simulink model "WaterProp"  (Simulink 7.9)
settings: Solver=FixedStepDiscrete  StartTime=0.0  StopTime=stop  FixedStep=1  MaxStep=1  RelTol=1e-3
settings Model: Creator=awohlfei  LastModifiedBy=awohlfei
settings DataIOCC: SaveTime=off

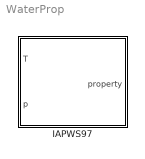
== system WaterProp ==
  IAPWS97 : Subsystem  mask{PROPERTY=DENSITY}
      mask StyleString: popup(DENSITY|HEAT_CAPACITY|THERMAL_CONDUCTIVITY|VISCOSITY|ENTHALPY|ENTROPY|PRANDTL|SPECIFIC_VOLUME|EVAPORATION_ENTHALPY|VAPOURPRESSURE|SATURATIONTEMPERATURE|SATURATIONPROPERTY|TEMPERATURE_CONDUCTIVITY|ENTHALPY2TEMPERATURE)

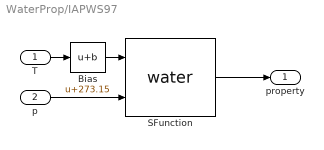
== system WaterProp/IAPWS97 ==
  T : Inport
  p : Inport  Port=2
  Bias : Bias  Bias=273.15
  SFunction : S-Function  FunctionName=water  Parameters=PROPERTY  EnableBusSupport=off
  property : Outport
  wires:
  T/1 -> Bias/1
  p/1 -> SFunction/2
  SFunction/1 -> property/1
  Bias/1 -> SFunction/1
